simulink model "dynamic_model_soft_robot"  (R2018a)
settings: Solver=ode4  StartTime=0.0  StopTime=t_span  FixedStep=dt  RelTol=1e-3
values from neighbouring files (symbols this model uses):
  alpha0 = 0    [data_simulate_srm_dynamic_model.m]
  c1 = 0.12    [data_simulate_srm_dynamic_model.m]
  c2 = 5.93e-7    (= 5.93e-07)    [data_simulate_srm_dynamic_model.m]
  c3 = 5.93e-7    (= 5.93e-07)    [data_simulate_srm_dynamic_model.m]
  d0 = 0.0644    [data_simulate_srm_dynamic_model.m]
  dq_0 = [0; 0; 500]    [data_simulate_srm_dynamic_model.m]
  dt = 1.00e-03    (= 0.001)    [data_simulate_srm_dynamic_model.m]    (also in simulateSoftRobot.m)
  g = 9.81    [data_simulate_srm_dynamic_model.m]    (also in simulateSoftRobot.m)
  m = 0.0494    [data_simulate_srm_dynamic_model.m]    (also in simulateSoftRobot.m)
  noise_ddq = 0*[1e-4, 1e-4, 1e-4]    [data_simulate_srm_dynamic_model.m]
  noise_dq = 0*[1e-4, 1e-4, 1e-4]    [data_simulate_srm_dynamic_model.m]
  noise_q = 0*[1e-6, 1e-1, 1e-1]    [data_simulate_srm_dynamic_model.m]
  p_true = [b1; b2; b3; b4; b5; b6]    [data_simulate_srm_dynamic_model.m]
  q_0 = [d0; 10; .1]    [data_simulate_srm_dynamic_model.m]
  r = 0.0235    [data_simulate_srm_dynamic_model.m]    (also in simulateSoftRobot.m = 0.02)
libraries: dspinverses x1
(part 2 of 3)

== matlab function dynamic_model_soft_robot/soft robotic manipulator dynamical model/Coreoilis matrix  ==
  data: q input; y output; dq input; m parameter; r parameter
function y = fcn(q,dq,m,r)

l = q(1);
kappa_x = q(2);
kappa_y1 = q(3);

dl = dq(1);
dkappa_x = dq(2);
dkappa_y = dq(3);

C = zeros(3,3);

C(1,1) = (dl*(4.0*m*sin(l*(kappa_x^2 + kappa_y1^2)^(1/2)) - 4.0*l*m*cos(l*(kappa_x^2 + kappa_y1^2)^(1/2))*(kappa_x^2 + kappa_y1^2)^(1/2)))/(2*l^2*(kappa_x^2 + kappa_y1^2)^(3/2)) - (2.0*dkappa_x*kappa_x*m*(3.0*kappa_x^2*l*(kappa_x^2 + kappa_y1^2)^(1/2) - 3.0*kappa_x^2*sin(l*(kappa_x^2 + kappa_y1^2)^(1/2)) - 3.0*kappa_y1^2*sin(l*(kappa_x^2 + kappa_y1^2)^(1/2)) - 1.0*l*(kappa_x^2 + kappa_y1^2)^(3/2) + 3.0*kappa_y1^2*l*(kappa_x^2 + kappa_y1^2)^(1/2) + kappa_x^2*l*cos(l*(kappa_x^2 + kappa_y1^2)^(1/2))*(kappa_x^2 + kappa_y1^2)^(1/2) + kappa_y1^2*l*cos(l*(kappa_x^2 + kappa_y1^2)^(1/2))*(kappa_x^2 + kappa_y1^2)^(1/2)))/(l*(kappa_x^2 + kappa_y1^2)^(7/2)) - (2.0*dkappa_y*kappa_y1*m*(3.0*kappa_x^2*l*(kappa_x^2 + kappa_y1^2)^(1/2) - 3.0*kappa_x^2*sin(l*(kappa_x^2 + kappa_y1^2)^(1/2)) - 3.0*kappa_y1^2*sin(l*(kappa_x^2 + kappa_y1^2)^(1/2)) - 1.0*l*(kappa_x^2 + kappa_y1^2)^(3/2) + 3.0*kappa_y1^2*l*(kappa_x^2 + kappa_y1^2)^(1/2) + kappa_x^2*l*cos(l*(kappa_x^2 + kappa_y1^2)^(1/2))*(kappa_x^2 + kappa_y1^2)^(1/2) + kappa_y1^2*l*cos(l*(kappa_x^2 + kappa_y1^2)^(1/2))*(kappa_x^2 + kappa_y1^2)^(1/2)))/(l*(kappa_x^2 + kappa_y1^2)^(7/2));
C(1,2) = - (dkappa_y*(4.0*kappa_x*kappa_y1*m*sin(l*(kappa_x^2 + kappa_y1^2)^(1/2)) + 0.5*kappa_x*kappa_y1*m*sin(2.0*l*(kappa_x^2 + kappa_y1^2)^(1/2)) - 2.0*kappa_x*kappa_y1^3*m*r^2*sin(l*(kappa_x^2 + kappa_y1^2)^(1/2)) - 2.0*kappa_x^3*kappa_y1*m*r^2*sin(l*(kappa_x^2 + kappa_y1^2)^(1/2)) + 60.0*kappa_x*kappa_y1*l*m*sin(l*(kappa_x^2 + kappa_y1^2)^(1/2)) + 0.125*kappa_x*kappa_y1^3*m*r^2*sin(2.0*l*(kappa_x^2 + kappa_y1^2)^(1/2)) + 0.125*kappa_x^3*kappa_y1*m*r^2*sin(2.0*l*(kappa_x^2 + kappa_y1^2)^(1/2)) - 32.0*kappa_x*kappa_y1*l^2*m*(kappa_x^2 + kappa_y1^2)^(1/2) + 1.3333333333333333333333333333333*kappa_x*kappa_y1*l^3*m*(kappa_x^2 + kappa_y1^2)^(3/2) - 1.0*kappa_x*kappa_y1*l*m*cos(2.0*l*(kappa_x^2 + kappa_y1^2)^(1/2))*(kappa_x^2 + kappa_y1^2)^(1/2) - 28.0*kappa_x*kappa_y1*l^2*m*cos(l*(kappa_x^2 + kappa_y1^2)^(1/2))*(kappa_x^2 + kappa_y1^2)^(1/2) - 4.0*kappa_x*kappa_y1*l*m*cos(l*(kappa_x^2 + kappa_y1^2)^(1/2))*(kappa_x^2 + kappa_y1^2)^(1/2) + 0.33333333333333333333333333333333*kappa_x*kappa_y1^3*l^3*m*r^2*(kappa_x^2 + kappa_y1^2)^(3/2) + 0.33333333333333333333333333333333*kappa_x^3*kappa_y1*l^3*m*r^2*(kappa_x^2 + kappa_y1^2)^(3/2) - 4.0*kappa_x*kappa_y1*l^2*m*sin(l*(kappa_x^2 + kappa_y1^2)^(1/2))*(kappa_x^2 + kappa_y1^2) - 4*kappa_x*kappa_y1*l^3*m*sin(l*(kappa_x^2 + kappa_y1^2)^(1/2))*(kappa_x^2 + kappa_y1^2) + 2.0*kappa_x*kappa_y1^3*l*m*r^2*cos(l*(kappa_x^2 + kappa_y1^2)^(1/2))*(kappa_x^2 + kappa_y1^2)^(1/2) + 2.0*kappa_x^3*kappa_y1*l*m*r^2*cos(l*(kappa_x^2 + kappa_y1^2)^(1/2))*(kappa_x^2 + kappa_y1^2)^(1/2) - 0.25*kappa_x*kappa_y1^3*l*m*r^2*cos(2.0*l*(kappa_x^2 + kappa_y1^2)^(1/2))*(kappa_x^2 + kappa_y1^2)^(1/2) - 0.25*kappa_x^3*kappa_y1*l*m*r^2*cos(2.0*l*(kappa_x^2 + kappa_y1^2)^(1/2))*(kappa_x^2 + kappa_y1^2)^(1/2)))/(2*l^2*(kappa_x^2 + kappa_y1^2)^(7/2)) - (dkappa_x*(8.0*kappa_x^2*m*sin(l*(kappa_x^2 + kappa_y1^2)^(1/2)) + 4.0*kappa_y1^2*m*sin(l*(kappa_x^2 + kappa_y1^2)^(1/2)) - 0.5*kappa_y1^2*m*sin(2.0*l*(kappa_x^2 + kappa_y1^2)^(1/2)) + 8.0*l^2*m*(kappa_x^2 + kappa_y1^2)^(3/2) - 0.125*kappa_y1^4*m*r^2*sin(2.0*l*(kappa_x^2 + kappa_y1^2)^(1/2)) + 4*l^2*m*cos(l*(kappa_x^2 + kappa_y1^2)^(1/2))*(kappa_x^2 + kappa_y1^2)^(3/2) + 60.0*kappa_x^2*l*m*sin(l*(kappa_x^2 + kappa_y1^2)^(1/2)) - 32.0*kappa_x^2*l^2*m*(kappa_x^2 + kappa_y1^2)^(1/2) + 1.3333333333333333333333333333333*kappa_x^2*l^3*m*(kappa_x^2 + kappa_y1^2)^(3/2) - 12.0*l*m*sin(l*(kappa_x^2 + kappa_y1^2)^(1/2))*(kappa_x^2 + kappa_y1^2) + 2.0*kappa_y1^4*m*r^2*sin(l*(kappa_x^2 + kappa_y1^2)^(1/2)) - 0.125*kappa_x^2*kappa_y1^2*m*r^2*sin(2.0*l*(kappa_x^2 + kappa_y1^2)^(1/2)) + kappa_y1^2*l*m*cos(2.0*l*(kappa_x^2 + kappa_y1^2)^(1/2))*(kappa_x^2 + kappa_y1^2)^(1/2) - 28.0*kappa_x^2*l^2*m*cos(l*(kappa_x^2 + kappa_y1^2)^(1/2))*(kappa_x^2 + kappa_y1^2)^(1/2) + 0.33333333333333333333333333333333*kappa_x^4*l^3*m*r^2*(kappa_x^2 + kappa_y1^2)^(3/2) + 2.0*kappa_x^2*kappa_y1^2*m*r^2*sin(l*(kappa_x^2 + kappa_y1^2)^(1/2)) - 8.0*kappa_x^2*l*m*cos(l*(kappa_x^2 + kappa_y1^2)^(1/2))*(kappa_x^2 + kappa_y1^2)^(1/2) - 4.0*kappa_y1^2*l*m*cos(l*(kappa_x^2 + kappa_y1^2)^(1/2))*(kappa_x^2 + kappa_y1^2)^(1/2) - 4.0*kappa_x^2*l^2*m*sin(l*(kappa_x^2 + kappa_y1^2)^(1/2))*(kappa_x^2 + kappa_y1^2) - 4*kappa_x^2*l^3*m*sin(l*(kappa_x^2 + kappa_y1^2)^(1/2))*(kappa_x^2 + kappa_y1^2) + 0.33333333333333333333333333333333*kappa_x^2*kappa_y1^2*l^3*m*r^2*(kappa_x^2 + kappa_y1^2)^(3/2) - 2.0*kappa_y1^4*l*m*r^2*cos(l*(kappa_x^2 + kappa_y1^2)^(1/2))*(kappa_x^2 + kappa_y1^2)^(1/2) + 0.25*kappa_y1^4*l*m*r^2*cos(2.0*l*(kappa_x^2 + kappa_y1^2)^(1/2))*(kappa_x^2 + kappa_y1^2)^(1/2) - 2.0*kappa_x^2*kappa_y1^2*l*m*r^2*cos(l*(kappa_x^2 + kappa_y1^2)^(1/2))*(kappa_x^2 + kappa_y1^2)^(1/2) + 0.25*kappa_x^2*kappa_y1^2*l*m*r^2*cos(2.0*l*(kappa_x^2 + kappa_y1^2)^(1/2))*(kappa_x^2 + kappa_y1^2)^(1/2)))/(2*l^2*(kappa_x^2 + kappa_y1^2)^(7/2)) - (2.0*dl*kappa_x*m*(3.0*kappa_x^2*l*(kappa_x^2 + kappa_y1^2)^(1/2) - 3.0*kappa_x^2*sin(l*(kappa_x^2 + kappa_y1^2)^(1/2)) - 3.0*kappa_y1^2*sin(l*(kappa_x^2 + kappa_y1^2)^(1/2)) - 1.0*l*(kappa_x^2 + kappa_y1^2)^(3/2) + 3.0*kappa_y1^2*l*(kappa_x^2 + kappa_y1^2)^(1/2) + kappa_x^2*l*cos(l*(kappa_x^2 + kappa_y1^2)^(1/2))*(kappa_x^2 + kappa_y1^2)^(1/2) + kappa_y1^2*l*cos(l*(kappa_x^2 + kappa_y1^2)^(1/2))*(kappa_x^2 + kappa_y1^2)^(1/2)))/(l*(kappa_x^2 + kappa_y1^2)^(7/2));
C(1,3) = - (dkappa_x*(4.0*kappa_x*kappa_y1*m*sin(l*(kappa_x^2 + kappa_y1^2)^(1/2)) + 0.5*kappa_x*kappa_y1*m*sin(2.0*l*(kappa_x^2 + kappa_y1^2)^(1/2)) - 2.0*kappa_x*kappa_y1^3*m*r^2*sin(l*(kappa_x^2 + kappa_y1^2)^(1/2)) - 2.0*kappa_x^3*kappa_y1*m*r^2*sin(l*(kappa_x^2 + kappa_y1^2)^(1/2)) + 60.0*kappa_x*kappa_y1*l*m*sin(l*(kappa_x^2 + kappa_y1^2)^(1/2)) + 0.125*kappa_x*kappa_y1^3*m*r^2*sin(2.0*l*(kappa_x^2 + kappa_y1^2)^(1/2)) + 0.125*kappa_x^3*kappa_y1*m*r^2*sin(2.0*l*(kappa_x^2 + kappa_y1^2)^(1/2)) - 32.0*kappa_x*kappa_y1*l^2*m*(kappa_x^2 + kappa_y1^2)^(1/2) + 1.3333333333333333333333333333333*kappa_x*kappa_y1*l^3*m*(kappa_x^2 + kappa_y1^2)^(3/2) - 1.0*kappa_x*kappa_y1*l*m*cos(2.0*l*(kappa_x^2 + kappa_y1^2)^(1/2))*(kappa_x^2 + kappa_y1^2)^(1/2) - 28.0*kappa_x*kappa_y1*l^2*m*cos(l*(kappa_x^2 + kappa_y1^2)^(1/2))*(kappa_x^2 + kappa_y1^2)^(1/2) - 4.0*kappa_x*kappa_y1*l*m*cos(l*(kappa_x^2 + kappa_y1^2)^(1/2))*(kappa_x^2 + kappa_y1^2)^(1/2) + 0.33333333333333333333333333333333*kappa_x*kappa_y1^3*l^3*m*r^2*(kappa_x^2 + kappa_y1^2)^(3/2) + 0.33333333333333333333333333333333*kappa_x^3*kappa_y1*l^3*m*r^2*(kappa_x^2 + kappa_y1^2)^(3/2) - 4.0*kappa_x*kappa_y1*l^2*m*sin(l*(kappa_x^2 + kappa_y1^2)^(1/2))*(kappa_x^2 + kappa_y1^2) - 4*kappa_x*kappa_y1*l^3*m*sin(l*(kappa_x^2 + kappa_y1^2)^(1/2))*(kappa_x^2 + kappa_y1^2) + 2.0*kappa_x*kappa_y1^3*l*m*r^2*cos(l*(kappa_x^2 + kappa_y1^2)^(1/2))*(kappa_x^2 + kappa_y1^2)^(1/2) + 2.0*kappa_x^3*kappa_y1*l*m*r^2*cos(l*(kappa_x^2 + kappa_y1^2)^(1/2))*(kappa_x^2 + kappa_y1^2)^(1/2) - 0.25*kappa_x*kappa_y1^3*l*m*r^2*cos(2.0*l*(kappa_x^2 + kappa_y1^2)^(1/2))*(kappa_x^2 + kappa_y1^2)^(1/2) - 0.25*kappa_x^3*kappa_y1*l*m*r^2*cos(2.0*l*(kappa_x^2 + kappa_y1^2)^(1/2))*(kappa_x^2 + kappa_y1^2)^(1/2)))/(2*l^2*(kappa_x^2 + kappa_y1^2)^(7/2)) - (dkappa_y*(4.0*kappa_x^2*m*sin(l*(kappa_x^2 + kappa_y1^2)^(1/2)) + 8.0*kappa_y1^2*m*sin(l*(kappa_x^2 + kappa_y1^2)^(1/2)) - 0.5*kappa_x^2*m*sin(2.0*l*(kappa_x^2 + kappa_y1^2)^(1/2)) + 8.0*l^2*m*(kappa_x^2 + kappa_y1^2)^(3/2) - 0.125*kappa_x^4*m*r^2*sin(2.0*l*(kappa_x^2 + kappa_y1^2)^(1/2)) + 4*l^2*m*cos(l*(kappa_x^2 + kappa_y1^2)^(1/2))*(kappa_x^2 + kappa_y1^2)^(3/2) + 60.0*kappa_y1^2*l*m*sin(l*(kappa_x^2 + kappa_y1^2)^(1/2)) - 32.0*kappa_y1^2*l^2*m*(kappa_x^2 + kappa_y1^2)^(1/2) + 1.3333333333333333333333333333333*kappa_y1^2*l^3*m*(kappa_x^2 + kappa_y1^2)^(3/2) - 12.0*l*m*sin(l*(kappa_x^2 + kappa_y1^2)^(1/2))*(kappa_x^2 + kappa_y1^2) + 2.0*kappa_x^4*m*r^2*sin(l*(kappa_x^2 + kappa_y1^2)^(1/2)) - 0.125*kappa_x^2*kappa_y1^2*m*r^2*sin(2.0*l*(kappa_x^2 + kappa_y1^2)^(1/2)) + kappa_x^2*l*m*cos(2.0*l*(kappa_x^2 + kappa_y1^2)^(1/2))*(kappa_x^2 + kappa_y1^2)^(1/2) - 28.0*kappa_y1^2*l^2*m*cos(l*(kappa_x^2 + kappa_y1^2)^(1/2))*(kappa_x^2 + kappa_y1^2)^(1/2) + 0.33333333333333333333333333333333*kappa_y1^4*l^3*m*r^2*(kappa_x^2 + kappa_y1^2)^(3/2) + 2.0*kappa_x^2*kappa_y1^2*m*r^2*sin(l*(kappa_x^2 + kappa_y1^2)^(1/2)) - 4.0*kappa_x^2*l*m*cos(l*(kappa_x^2 + kappa_y1^2)^(1/2))*(kappa_x^2 + kappa_y1^2)^(1/2) - 8.0*kappa_y1^2*l*m*cos(l*(kappa_x^2 + kappa_y1^2)^(1/2))*(kappa_x^2 + kappa_y1^2)^(1/2) - 4.0*kappa_y1^2*l^2*m*sin(l*(kappa_x^2 + kappa_y1^2)^(1/2))*(kappa_x^2 + kappa_y1^2) - 4*kappa_y1^2*l^3*m*sin(l*(kappa_x^2 + kappa_y1^2)^(1/2))*(kappa_x^2 + kappa_y1^2) + 0.33333333333333333333333333333333*kappa_x^2*kappa_y1^2*l^3*m*r^2*(kappa_x^2 + kappa_y1^2)^(3/2) - 2.0*kappa_x^4*l*m*r^2*cos(l*(kappa_x^2 + kappa_y1^2)^(1/2))*(kappa_x^2 + kappa_y1^2)^(1/2) + 0.25*kappa_x^4*l*m*r^2*cos(2.0*l*(kappa_x^2 + kappa_y1^2)^(1/2))*(kappa_x^2 + kappa_y1^2)^(1/2) - 2.0*kappa_x^2*kappa_y1^2*l*m*r^2*cos(l*(kappa_x^2 + kappa_y1^2)^(1/2))*(kappa_x^2 + kappa_y1^2)^(1/2) + 0.25*kappa_x^2*kappa_y1^2*l*m*r^2*cos(2.0*l*(kappa_x^2 + kappa_y1^2)^(1/2))*(kappa_x^2 + kappa_y1^2)^(1/2)))/(2*l^2*(kappa_x^2 + kappa_y1^2)^(7/2)) - (2.0*dl*kappa_y1*m*(3.0*kappa_x^2*l*(kappa_x^2 + kappa_y1^2)^(1/2) - 3.0*kappa_x^2*sin(l*(kappa_x^2 + kappa_y1^2)^(1/2)) - 3.0*kappa_y1^2*sin(l*(kappa_x^2 + kappa_y1^2)^(1/2)) - 1.0*l*(kappa_x^2 + kappa_y1^2)^(3/2) + 3.0*kappa_y1^2*l*(kappa_x^2 + kappa_y1^2)^(1/2) + kappa_x^2*l*cos(l*(kappa_x^2 + kappa_y1^2)^(1/2))*(kappa_x^2 + kappa_y1^2)^(1/2) + kappa_y1^2*l*cos(l*(kappa_x^2 + kappa_y1^2)^(1/2))*(kappa_x^2 + kappa_y1^2)^(1/2)))/(l*(kappa_x^2 + kappa_y1^2)^(7/2));

C(2,1) = (dkappa_y*(4.0*kappa_x*kappa_y1*m*sin(l*(kappa_x^2 + kappa_y1^2)^(1/2)) + 0.5*kappa_x*kappa_y1*m*sin(2.0*l*(kappa_x^2 + kappa_y1^2)^(1/2)) - 2.0*kappa_x*kappa_y1^3*m*r^2*sin(l*(kappa_x^2 + kappa_y1^2)^(1/2)) - 2.0*kappa_x^3*kappa_y1*m*r^2*sin(l*(kappa_x^2 + kappa_y1^2)^(1/2)) + 0.125*kappa_x*kappa_y1^3*m*r^2*sin(2.0*l*(kappa_x^2 + kappa_y1^2)^(1/2)) + 0.125*kappa_x^3*kappa_y1*m*r^2*sin(2.0*l*(kappa_x^2 + kappa_y1^2)^(1/2)) + 1.3333333333333333333333333333333*kappa_x*kappa_y1*l^3*m*(kappa_x^2 + kappa_y1^2)^(3/2) - 1.0*kappa_x*kappa_y1*l*m*cos(2.0*l*(kappa_x^2 + kappa_y1^2)^(1/2))*(kappa_x^2 + kappa_y1^2)^(1/2) - 4.0*kappa_x*kappa_y1*l*m*cos(l*(kappa_x^2 + kappa_y1^2)^(1/2))*(kappa_x^2 + kappa_y1^2)^(1/2) + 0.33333333333333333333333333333333*kappa_x*kappa_y1^3*l^3*m*r^2*(kappa_x^2 + kappa_y1^2)^(3/2) + 0.33333333333333333333333333333333*kappa_x^3*kappa_y1*l^3*m*r^2*(kappa_x^2 + kappa_y1^2)^(3/2) - 4.0*kappa_x*kappa_y1*l^2*m*sin(l*(kappa_x^2 + kappa_y1^2)^(1/2))*(kappa_x^2 + kappa_y1^2) + 2.0*kappa_x*kappa_y1^3*l*m*r^2*cos(l*(kappa_x^2 + kappa_y1^2)^(1/2))*(kappa_x^2 + kappa_y1^2)^(1/2) + 2.0*kappa_x^3*kappa_y1*l*m*r^2*cos(l*(kappa_x^2 + kappa_y1^2)^(1/2))*(kappa_x^2 + kappa_y1^2)^(1/2) - 0.25*kappa_x*kappa_y1^3*l*m*r^2*cos(2.0*l*(kappa_x^2 + kappa_y1^2)^(1/2))*(kappa_x^2 + kappa_y1^2)^(1/2) - 0.25*kappa_x^3*kappa_y1*l*m*r^2*cos(2.0*l*(kappa_x^2 + kappa_y1^2)^(1/2))*(kappa_x^2 + kappa_y1^2)^(1/2)))/(2*l^2*(kappa_x^2 + kappa_y1^2)^(7/2)) + (dkappa_x*(8.0*kappa_x^2*m*sin(l*(kappa_x^2 + kappa_y1^2)^(1/2)) + 4.0*kappa_y1^2*m*sin(l*(kappa_x^2 + kappa_y1^2)^(1/2)) - 0.5*kappa_y1^2*m*sin(2.0*l*(kappa_x^2 + kappa_y1^2)^(1/2)) - 0.125*kappa_y1^4*m*r^2*sin(2.0*l*(kappa_x^2 + kappa_y1^2)^(1/2)) + 1.3333333333333333333333333333333*kappa_x^2*l^3*m*(kappa_x^2 + kappa_y1^2)^(3/2) + 2.0*kappa_y1^4*m*r^2*sin(l*(kappa_x^2 + kappa_y1^2)^(1/2)) - 0.125*kappa_x^2*kappa_y1^2*m*r^2*sin(2.0*l*(kappa_x^2 + kappa_y1^2)^(1/2)) + kappa_y1^2*l*m*cos(2.0*l*(kappa_x^2 + kappa_y1^2)^(1/2))*(kappa_x^2 + kappa_y1^2)^(1/2) + 0.33333333333333333333333333333333*kappa_x^4*l^3*m*r^2*(kappa_x^2 + kappa_y1^2)^(3/2) + 2.0*kappa_x^2*kappa_y1^2*m*r^2*sin(l*(kappa_x^2 + kappa_y1^2)^(1/2)) - 8.0*kappa_x^2*l*m*cos(l*(kappa_x^2 + kappa_y1^2)^(1/2))*(kappa_x^2 + kappa_y1^2)^(1/2) - 4.0*kappa_y1^2*l*m*cos(l*(kappa_x^2 + kappa_y1^2)^(1/2))*(kappa_x^2 + kappa_y1^2)^(1/2) - 4.0*kappa_x^2*l^2*m*sin(l*(kappa_x^2 + kappa_y1^2)^(1/2))*(kappa_x^2 + kappa_y1^2) + 0.33333333333333333333333333333333*kappa_x^2*kappa_y1^2*l^3*m*r^2*(kappa_x^2 + kappa_y1^2)^(3/2) - 2.0*kappa_y1^4*l*m*r^2*cos(l*(kappa_x^2 + kappa_y1^2)^(1/2))*(kappa_x^2 + kappa_y1^2)^(1/2) + 0.25*kappa_y1^4*l*m*r^2*cos(2.0*l*(kappa_x^2 + kappa_y1^2)^(1/2))*(kappa_x^2 + kappa_y1^2)^(1/2) - 2.0*kappa_x^2*kappa_y1^2*l*m*r^2*cos(l*(kappa_x^2 + kappa_y1^2)^(1/2))*(kappa_x^2 + kappa_y1^2)^(1/2) + 0.25*kappa_x^2*kappa_y1^2*l*m*r^2*cos(2.0*l*(kappa_x^2 + kappa_y1^2)^(1/2))*(kappa_x^2 + kappa_y1^2)^(1/2)))/(2*l^2*(kappa_x^2 + kappa_y1^2)^(7/2)) + (dl*(12.0*kappa_x^3*l^2*m*(kappa_x^2 + kappa_y1^2)^(1/2) - 20.0*kappa_x^3*l*m*sin(l*(kappa_x^2 + kappa_y1^2)^(1/2)) - 4.0*kappa_x*l^2*m*(kappa_x^2 + kappa_y1^2)^(3/2) - 12.0*kappa_x*m*sin(l*(kappa_x^2 + kappa_y1^2)^(1/2))*(kappa_x^2 + kappa_y1^2) - 20.0*kappa_x*kappa_y1^2*l*m*sin(l*(kappa_x^2 + kappa_y1^2)^(1/2)) + 12.0*kappa_x*kappa_y1^2*l^2*m*(kappa_x^2 + kappa_y1^2)^(1/2) + 8.0*kappa_x*l*m*sin(l*(kappa_x^2 + kappa_y1^2)^(1/2))*(kappa_x^2 + kappa_y1^2) + 4.0*kappa_x^3*l^2*m*cos(l*(kappa_x^2 + kappa_y1^2)^(1/2))*(kappa_x^2 + kappa_y1^2)^(1/2) + 12.0*kappa_x*l*m*cos(l*(kappa_x^2 + kappa_y1^2)^(1/2))*(kappa_x^2 + kappa_y1^2)^(3/2) + 4*kappa_x*l^2*m*sin(l*(kappa_x^2 + kappa_y1^2)^(1/2))*(kappa_x^2 + kappa_y1^2)^2 + 4.0*kappa_x*kappa_y1^2*l^2*m*cos(l*(kappa_x^2 + kappa_y1^2)^(1/2))*(kappa_x^2 + kappa_y1^2)^(1/2)))/(2*l^2*(kappa_x^2 + kappa_y1^2)^(7/2));
C(2,2) = (dl*(8.0*kappa_x^2*m*sin(l*(kappa_x^2 + kappa_y1^2)^(1/2)) + 4.0*kappa_y1^2*m*sin(l*(kappa_x^2 + kappa_y1^2)^(1/2)) - 0.5*kappa_y1^2*m*sin(2.0*l*(kappa_x^2 + kappa_y1^2)^(1/2)) - 0.125*kappa_y1^4*m*r^2*sin(2.0*l*(kappa_x^2 + kappa_y1^2)^(1/2)) + 1.3333333333333333333333333333333*kappa_x^2*l^3*m*(kappa_x^2 + kappa_y1^2)^(3/2) + 2.0*kappa_y1^4*m*r^2*sin(l*(kappa_x^2 + kappa_y1^2)^(1/2)) - 0.125*kappa_x^2*kappa_y1^2*m*r^2*sin(2.0*l*(kappa_x^2 + kappa_y1^2)^(1/2)) + kappa_y1^2*l*m*cos(2.0*l*(kappa_x^2 + kappa_y1^2)^(1/2))*(kappa_x^2 + kappa_y1^2)^(1/2) + 0.33333333333333333333333333333333*kappa_x^4*l^3*m*r^2*(kappa_x^2 + kappa_y1^2)^(3/2) + 2.0*kappa_x^2*kappa_y1^2*m*r^2*sin(l*(kappa_x^2 + kappa_y1^2)^(1/2)) - 8.0*kappa_x^2*l*m*cos(l*(kappa_x^2 + kappa_y1^2)^(1/2))*(kappa_x^2 + kappa_y1^2)^(1/2) - 4.0*kappa_y1^2*l*m*cos(l*(kappa_x^2 + kappa_y1^2)^(1/2))*(kappa_x^2 + kappa_y1^2)^(1/2) - 4.0*kappa_x^2*l^2*m*sin(l*(kappa_x^2 + kappa_y1^2)^(1/2))*(kappa_x^2 + kappa_y1^2) + 0.33333333333333333333333333333333*kappa_x^2*kappa_y1^2*l^3*m*r^2*(kappa_x^2 + kappa_y1^2)^(3/2) - 2.0*kappa_y1^4*l*m*r^2*cos(l*(kappa_x^2 + kappa_y1^2)^(1/2))*(kappa_x^2 + kappa_y1^2)^(1/2) + 0.25*kappa_y1^4*l*m*r^2*cos(2.0*l*(kappa_x^2 + kappa_y1^2)^(1/2))*(kappa_x^2 + kappa_y1^2)^(1/2) - 2.0*kappa_x^2*kappa_y1^2*l*m*r^2*cos(l*(kappa_x^2 + kappa_y1^2)^(1/2))*(kappa_x^2 + kappa_y1^2)^(1/2) + 0.25*kappa_x^2*kappa_y1^2*l*m*r^2*cos(2.0*l*(kappa_x^2 + kappa_y1^2)^(1/2))*(kappa_x^2 + kappa_y1^2)^(1/2)))/(2*l^2*(kappa_x^2 + kappa_y1^2)^(7/2)) - (5.0e-34*dkappa_y*(2.5e33*kappa_y1^3*m*sin(2.0*l*(kappa_x^2 + kappa_y1^2)^(1/2)) - 2.0e34*kappa_y1^3*m*sin(l*(kappa_x^2 + kappa_y1^2)^(1/2)) + 375000000000000000000000000000000.0*kappa_y1^5*m*r^2*sin(2.0*l*(kappa_x^2 + kappa_y1^2)^(1/2)) - 4.8e34*kappa_x^2*kappa_y1*m*sin(l*(kappa_x^2 + kappa_y1^2)^(1/2)) - 1.0e33*kappa_x^2*kappa_y1*m*sin(2.0*l*(kappa_x^2 + kappa_y1^2)^(1/2)) + 1.2e34*kappa_y1*l*m*(kappa_x^2 + kappa_y1^2)^(3/2) - 6.0e33*kappa_y1^5*m*r^2*sin(l*(kappa_x^2 + kappa_y1^2)^(1/2)) + 125000000000000000000000000000000.0*kappa_x^2*kappa_y1^3*m*r^2*sin(2.0*l*(kappa_x^2 + kappa_y1^2)^(1/2)) - 1.0e33*kappa_y1^3*l*m*cos(2.0*l*(kappa_x^2 + kappa_y1^2)^(1/2))*(kappa_x^2 + kappa_y1^2)^(1/2) + 2.6666666666666666666666666666667e33*kappa_x^2*kappa_y1*l^3*m*(kappa_x^2 + kappa_y1^2)^(3/2) + 5.0e33*kappa_y1^3*l*m*r^2*(kappa_x^2 + kappa_y1^2)^(3/2) + 1.5e33*kappa_y1^5*l*m*r^2*(kappa_x^2 + kappa_y1^2)^(1/2) + 4.0e33*kappa_x^4*kappa_y1*l^2*m*sin(l*(kappa_x^2 + kappa_y1^2)^(1/2)) + 4.0e33*kappa_x^4*kappa_y1*m*r^2*sin(l*(kappa_x^2 + kappa_y1^2)^(1/2)) - 250000000000000000000000000000000.0*kappa_x^4*kappa_y1*m*r^2*sin(2.0*l*(kappa_x^2 + kappa_y1^2)^(1/2)) + 4.0e33*kappa_x^2*kappa_y1^3*l^2*m*sin(l*(kappa_x^2 + kappa_y1^2)^(1/2)) + 6.0e33*kappa_x^2*kappa_y1*l*m*(kappa_x^2 + kappa_y1^2)^(1/2) - 2.0e33*kappa_x^2*kappa_y1^3*m*r^2*sin(l*(kappa_x^2 + kappa_y1^2)^(1/2)) - 3.0e33*kappa_y1*l*m*r^2*(kappa_x^2 + kappa_y1^2)^(5/2) + 4.0e33*kappa_y1^3*l*m*cos(l*(kappa_x^2 + kappa_y1^2)^(1/2))*(kappa_x^2 + kappa_y1^2)^(1/2) + 3.2e34*kappa_x^2*kappa_y1*l*m*cos(l*(kappa_x^2 + kappa_y1^2)^(1/2))*(kappa_x^2 + kappa_y1^2)^(1/2) + 666666666666666666666666666666677.0*kappa_x^2*kappa_y1^3*l^3*m*r^2*(kappa_x^2 + kappa_y1^2)^(3/2) - 500000000000000000000000000000000.0*kappa_x^2*kappa_y1*l*m*r^2*(kappa_x^2 + kappa_y1^2)^(3/2) + 2.0e33*kappa_y1^5*l*m*r^2*cos(l*(kappa_x^2 + kappa_y1^2)^(1/2))*(kappa_x^2 + kappa_y1^2)^(1/2) - 250000000000000000000000000000000.0*kappa_y1^5*l*m*r^2*cos(2.0*l*(kappa_x^2 + kappa_y1^2)^(1/2))*(kappa_x^2 + kappa_y1^2)^(1/2) + 1.5e33*kappa_x^2*kappa_y1^3*l*m*r^2*(kappa_x^2 + kappa_y1^2)^(1/2) - 333333333333333333333333333333333.0*kappa_x^2*kappa_y1*l^3*m*r^2*(kappa_x^2 + kappa_y1^2)^(5/2) + 666666666666666666666666666666677.0*kappa_x^4*kappa_y1*l^3*m*r^2*(kappa_x^2 + kappa_y1^2)^(3/2) + 2.0e33*kappa_x^2*kappa_y1^3*l*m*r^2*cos(l*(kappa_x^2 + kappa_y1^2)^(1/2))*(kappa_x^2 + kappa_y1^2)^(1/2) - 250000000000000000000000000000000.0*kappa_x^2*kappa_y1^3*l*m*r^2*cos(2.0*l*(kappa_x^2 + kappa_y1^2)^(1/2))*(kappa_x^2 + kappa_y1^2)^(1/2)))/(l*(kappa_x^2 + kappa_y1^2)^(9/2)) - (5.0e-34*dkappa_x*(6.0e33*kappa_x^3*l*m*(kappa_x^2 + kappa_y1^2)^(1/2) - 4.0e34*kappa_x^3*m*sin(l*(kappa_x^2 + kappa_y1^2)^(1/2)) - 1.3333333333333333333333333333333e33*kappa_x*l^3*m*(kappa_x^2 + kappa_y1^2)^(5/2) - 1.2e34*kappa_x*kappa_y1^2*m*sin(l*(kappa_x^2 + kappa_y1^2)^(1/2)) + 2.6666666666666666666666666666667e33*kappa_x^3*l^3*m*(kappa_x^2 + kappa_y1^2)^(3/2) + 3.5e33*kappa_x*kappa_y1^2*m*sin(2.0*l*(kappa_x^2 + kappa_y1^2)^(1/2)) + 4.0e33*kappa_x^5*l^2*m*sin(l*(kappa_x^2 + kappa_y1^2)^(1/2)) + 1.0e34*kappa_x*l*m*(kappa_x^2 + kappa_y1^2)^(3/2) + 625000000000000000000000000000000.0*kappa_x^3*kappa_y1^2*m*r^2*sin(2.0*l*(kappa_x^2 + kappa_y1^2)^(1/2)) - 1.0e34*kappa_x*kappa_y1^4*m*r^2*sin(l*(kappa_x^2 + kappa_y1^2)^(1/2)) - 8.0e33*kappa_x*l*m*cos(l*(kappa_x^2 + kappa_y1^2)^(1/2))*(kappa_x^2 + kappa_y1^2)^(3/2) - 666666666666666666666666666666677.0*kappa_x^3*l^3*m*r^2*(kappa_x^2 + kappa_y1^2)^(5/2) + 666666666666666666666666666666677.0*kappa_x^5*l^3*m*r^2*(kappa_x^2 + kappa_y1^2)^(3/2) + 625000000000000000000000000000000.0*kappa_x*kappa_y1^4*m*r^2*sin(2.0*l*(kappa_x^2 + kappa_y1^2)^(1/2)) + 4.0e33*kappa_x^3*kappa_y1^2*l^2*m*sin(l*(kappa_x^2 + kappa_y1^2)^(1/2)) - 1.0e34*kappa_x^3*kappa_y1^2*m*r^2*sin(l*(kappa_x^2 + kappa_y1^2)^(1/2)) + 3.2e34*kappa_x^3*l*m*cos(l*(kappa_x^2 + kappa_y1^2)^(1/2))*(kappa_x^2 + kappa_y1^2)^(1/2) + 4.0e33*kappa_x*kappa_y1^2*l*m*cos(l*(kappa_x^2 + kappa_y1^2)^(1/2))*(kappa_x^2 + kappa_y1^2)^(1/2) + 666666666666666666666666666666677.0*kappa_x^3*kappa_y1^2*l^3*m*r^2*(kappa_x^2 + kappa_y1^2)^(3/2) - 1.0e33*kappa_x*kappa_y1^2*l*m*cos(2.0*l*(kappa_x^2 + kappa_y1^2)^(1/2))*(kappa_x^2 + kappa_y1^2)^(1/2) + 5.5e33*kappa_x*kappa_y1^2*l*m*r^2*(kappa_x^2 + kappa_y1^2)^(3/2) + 1.5e33*kappa_x*kappa_y1^4*l*m*r^2*(kappa_x^2 + kappa_y1^2)^(1/2) + 1.5e33*kappa_x^3*kappa_y1^2*l*m*r^2*(kappa_x^2 + kappa_y1^2)^(1/2) - 333333333333333333333333333333333.0*kappa_x*kappa_y1^2*l^3*m*r^2*(kappa_x^2 + kappa_y1^2)^(5/2) + 2.0e33*kappa_x*kappa_y1^4*l*m*r^2*cos(l*(kappa_x^2 + kappa_y1^2)^(1/2))*(kappa_x^2 + kappa_y1^2)^(1/2) - 250000000000000000000000000000000.0*kappa_x*kappa_y1^4*l*m*r^2*cos(2.0*l*(kappa_x^2 + kappa_y1^2)^(1/2))*(kappa_x^2 + kappa_y1^2)^(1/2) + 2.0e33*kappa_x^3*kappa_y1^2*l*m*r^2*cos(l*(kappa_x^2 + kappa_y1^2)^(1/2))*(kappa_x^2 + kappa_y1^2)^(1/2) - 250000000000000000000000000000000.0*kappa_x^3*kappa_y1^2*l*m*r^2*cos(2.0*l*(kappa_x^2 + kappa_y1^2)^(1/2))*(kappa_x^2 + kappa_y1^2)^(1/2)))/(l*(kappa_x^2 + kappa_y1^2)^(9/2));
C(2,3) = (dkappa_y*(1.5*kappa_x^3*m*sin(2.0*l*(kappa_x^2 + kappa_y1^2)^(1/2)) - 28.0*kappa_x^3*m*sin(l*(kappa_x^2 + kappa_y1^2)^(1/2)) + 0.125*kappa_x^5*m*r^2*sin(2.0*l*(kappa_x^2 + kappa_y1^2)^(1/2)) + 1.3333333333333333333333333333333*kappa_x*l^3*m*(kappa_x^2 + kappa_y1^2)^(5/2) + 5.0*kappa_x*kappa_y1^2*m*sin(2.0*l*(kappa_x^2 + kappa_y1^2)^(1/2)) + 14.0*kappa_x*l*m*(kappa_x^2 + kappa_y1^2)^(3/2) - 2.0*kappa_x^5*m*r^2*sin(l*(kappa_x^2 + kappa_y1^2)^(1/2)) + 0.875*kappa_x^3*kappa_y1^2*m*r^2*sin(2.0*l*(kappa_x^2 + kappa_y1^2)^(1/2)) - 1.0*kappa_x^3*l*m*cos(2.0*l*(kappa_x^2 + kappa_y1^2)^(1/2))*(kappa_x^2 + kappa_y1^2)^(1/2) - 2.6666666666666666666666666666667*kappa_x*kappa_y1^2*l^3*m*(kappa_x^2 + kappa_y1^2)^(3/2) + 4.5*kappa_x^3*l*m*r^2*(kappa_x^2 + kappa_y1^2)^(3/2) + 1.5*kappa_x^5*l*m*r^2*(kappa_x^2 + kappa_y1^2)^(1/2) - 4.0*kappa_x*kappa_y1^4*l^2*m*sin(l*(kappa_x^2 + kappa_y1^2)^(1/2)) - 12.0*kappa_x*kappa_y1^4*m*r^2*sin(l*(kappa_x^2 + kappa_y1^2)^(1/2)) + 8.0*kappa_x*l*m*cos(l*(kappa_x^2 + kappa_y1^2)^(1/2))*(kappa_x^2 + kappa_y1^2)^(3/2) + 0.33333333333333333333333333333333*kappa_x^3*l^3*m*r^2*(kappa_x^2 + kappa_y1^2)^(5/2) + 0.75*kappa_x*kappa_y1^4*m*r^2*sin(2.0*l*(kappa_x^2 + kappa_y1^2)^(1/2)) - 4.0*kappa_x^3*kappa_y1^2*l^2*m*sin(l*(kappa_x^2 + kappa_y1^2)^(1/2)) - 6.0*kappa_x*kappa_y1^2*l*m*(kappa_x^2 + kappa_y1^2)^(1/2) - 14.0*kappa_x^3*kappa_y1^2*m*r^2*sin(l*(kappa_x^2 + kappa_y1^2)^(1/2)) - 6.0*kappa_x*l*m*r^2*(kappa_x^2 + kappa_y1^2)^(5/2) + 4.0*kappa_x^3*l*m*cos(l*(kappa_x^2 + kappa_y1^2)^(1/2))*(kappa_x^2 + kappa_y1^2)^(1/2) - 24.0*kappa_x*kappa_y1^2*l*m*cos(l*(kappa_x^2 + kappa_y1^2)^(1/2))*(kappa_x^2 + kappa_y1^2)^(1/2) - 0.66666666666666666666666666666667*kappa_x^3*kappa_y1^2*l^3*m*r^2*(kappa_x^2 + kappa_y1^2)^(3/2) - 2.0*kappa_x*kappa_y1^2*l*m*cos(2.0*l*(kappa_x^2 + kappa_y1^2)^(1/2))*(kappa_x^2 + kappa_y1^2)^(1/2) + 10.0*kappa_x*kappa_y1^2*l*m*r^2*(kappa_x^2 + kappa_y1^2)^(3/2) + 3.0*kappa_x*kappa_y1^4*l*m*r^2*(kappa_x^2 + kappa_y1^2)^(1/2) + 2.0*kappa_x^5*l*m*r^2*cos(l*(kappa_x^2 + kappa_y1^2)^(1/2))*(kappa_x^2 + kappa_y1^2)^(1/2) - 0.25*kappa_x^5*l*m*r^2*cos(2.0*l*(kappa_x^2 + kappa_y1^2)^(1/2))*(kappa_x^2 + kappa_y1^2)^(1/2) + 4.5*kappa_x^3*kappa_y1^2*l*m*r^2*(kappa_x^2 + kappa_y1^2)^(1/2) + 0.66666666666666666666666666666667*kappa_x*kappa_y1^2*l^3*m*r^2*(kappa_x^2 + kappa_y1^2)^(5/2) - 0.66666666666666666666666666666667*kappa_x*kappa_y1^4*l^3*m*r^2*(kappa_x^2 + kappa_y1^2)^(3/2) + 4.0*kappa_x*kappa_y1^4*l*m*r^2*cos(l*(kappa_x^2 + kappa_y1^2)^(1/2))*(kappa_x^2 + kappa_y1^2)^(1/2) - 0.5*kappa_x*kappa_y1^4*l*m*r^2*cos(2.0*l*(kappa_x^2 + kappa_y1^2)^(1/2))*(kappa_x^2 + kappa_y1^2)^(1/2) + 6.0*kappa_x^3*kappa_y1^2*l*m*r^2*cos(l*(kappa_x^2 + kappa_y1^2)^(1/2))*(kappa_x^2 + kappa_y1^2)^(1/2) - 0.75*kappa_x^3*kappa_y1^2*l*m*r^2*cos(2.0*l*(kappa_x^2 + kappa_y1^2)^(1/2))*(kappa_x^2 + kappa_y1^2)^(1/2)))/(2*l*(kappa_x^2 + kappa_y1^2)^(9/2)) - (5.0e-34*dkappa_x*(2.5e33*kappa_y1^3*m*sin(2.0*l*(kappa_x^2 + kappa_y1^2)^(1/2)) - 2.0e34*kappa_y1^3*m*sin(l*(kappa_x^2 + kappa_y1^2)^(1/2)) + 375000000000000000000000000000000.0*kappa_y1^5*m*r^2*sin(2.0*l*(kappa_x^2 + kappa_y1^2)^(1/2)) - 4.8e34*kappa_x^2*kappa_y1*m*sin(l*(kappa_x^2 + kappa_y1^2)^(1/2)) - 1.0e33*kappa_x^2*kappa_y1*m*sin(2.0*l*(kappa_x^2 + kappa_y1^2)^(1/2)) + 1.2e34*kappa_y1*l*m*(kappa_x^2 + kappa_y1^2)^(3/2) - 6.0e33*kappa_y1^5*m*r^2*sin(l*(kappa_x^2 + kappa_y1^2)^(1/2)) + 125000000000000000000000000000000.0*kappa_x^2*kappa_y1^3*m*r^2*sin(2.0*l*(kappa_x^2 + kappa_y1^2)^(1/2)) - 1.0e33*kappa_y1^3*l*m*cos(2.0*l*(kappa_x^2 + kappa_y1^2)^(1/2))*(kappa_x^2 + kappa_y1^2)^(1/2) + 2.6666666666666666666666666666667e33*kappa_x^2*kappa_y1*l^3*m*(kappa_x^2 + kappa_y1^2)^(3/2) + 5.0e33*kappa_y1^3*l*m*r^2*(kappa_x^2 + kappa_y1^2)^(3/2) + 1.5e33*kappa_y1^5*l*m*r^2*(kappa_x^2 + kappa_y1^2)^(1/2) + 4.0e33*kappa_x^4*kappa_y1*l^2*m*sin(l*(kappa_x^2 + kappa_y1^2)^(1/2)) + 4.0e33*kappa_x^4*kappa_y1*m*r^2*sin(l*(kappa_x^2 + kappa_y1^2)^(1/2)) - 250000000000000000000000000000000.0*kappa_x^4*kappa_y1*m*r^2*sin(2.0*l*(kappa_x^2 + kappa_y1^2)^(1/2)) + 4.0e33*kappa_x^2*kappa_y1^3*l^2*m*sin(l*(kappa_x^2 + kappa_y1^2)^(1/2)) + 6.0e33*kappa_x^2*kappa_y1*l*m*(kappa_x^2 + kappa_y1^2)^(1/2) - 2.0e33*kappa_x^2*kappa_y1^3*m*r^2*sin(l*(kappa_x^2 + kappa_y1^2)^(1/2)) - 3.0e33*kappa_y1*l*m*r^2*(kappa_x^2 + kappa_y1^2)^(5/2) + 4.0e33*kappa_y1^3*l*m*cos(l*(kappa_x^2 + kappa_y1^2)^(1/2))*(kappa_x^2 + kappa_y1^2)^(1/2) + 3.2e34*kappa_x^2*kappa_y1*l*m*cos(l*(kappa_x^2 + kappa_y1^2)^(1/2))*(kappa_x^2 + kappa_y1^2)^(1/2) + 666666666666666666666666666666677.0*kappa_x^2*kappa_y1^3*l^3*m*r^2*(kappa_x^2 + kappa_y1^2)^(3/2) - 500000000000000000000000000000000.0*kappa_x^2*kappa_y1*l*m*r^2*(kappa_x^2 + kappa_y1^2)^(3/2) + 2.0e33*kappa_y1^5*l*m*r^2*cos(l*(kappa_x^2 + kappa_y1^2)^(1/2))*(kappa_x^2 + kappa_y1^2)^(1/2) - 250000000000000000000000000000000.0*kappa_y1^5*l*m*r^2*cos(2.0*l*(kappa_x^2 + kappa_y1^2)^(1/2))*(kappa_x^2 + kappa_y1^2)^(1/2) + 1.5e33*kappa_x^2*kappa_y1^3*l*m*r^2*(kappa_x^2 + kappa_y1^2)^(1/2) - 333333333333333333333333333333333.0*kappa_x^2*kappa_y1*l^3*m*r^2*(kappa_x^2 + kappa_y1^2)^(5/2) + 666666666666666666666666666666677.0*kappa_x^4*kappa_y1*l^3*m*r^2*(kappa_x^2 + kappa_y1^2)^(3/2) + 2.0e33*kappa_x^2*kappa_y1^3*l*m*r^2*cos(l*(kappa_x^2 + kappa_y1^2)^(1/2))*(kappa_x^2 + kappa_y1^2)^(1/2) - 250000000000000000000000000000000.0*kappa_x^2*kappa_y1^3*l*m*r^2*cos(2.0*l*(kappa_x^2 + kappa_y1^2)^(1/2))*(kappa_x^2 + kappa_y1^2)^(1/2)))/(l*(kappa_x^2 + kappa_y1^2)^(9/2)) + (dl*(4.0*kappa_x*kappa_y1*m*sin(l*(kappa_x^2 + kappa_y1^2)^(1/2)) + 0.5*kappa_x*kappa_y1*m*sin(2.0*l*(kappa_x^2 + kappa_y1^2)^(1/2)) - 2.0*kappa_x*kappa_y1^3*m*r^2*sin(l*(kappa_x^2 + kappa_y1^2)^(1/2)) - 2.0*kappa_x^3*kappa_y1*m*r^2*sin(l*(kappa_x^2 + kappa_y1^2)^(1/2)) + 0.125*kappa_x*kappa_y1^3*m*r^2*sin(2.0*l*(kappa_x^2 + kappa_y1^2)^(1/2)) + 0.125*kappa_x^3*kappa_y1*m*r^2*sin(2.0*l*(kappa_x^2 + kappa_y1^2)^(1/2)) + 1.3333333333333333333333333333333*kappa_x*kappa_y1*l^3*m*(kappa_x^2 + kappa_y1^2)^(3/2) - 1.0*kappa_x*kappa_y1*l*m*cos(2.0*l*(kappa_x^2 + kappa_y1^2)^(1/2))*(kappa_x^2 + kappa_y1^2)^(1/2) - 4.0*kappa_x*kappa_y1*l*m*cos(l*(kappa_x^2 + kappa_y1^2)^(1/2))*(kappa_x^2 + kappa_y1^2)^(1/2) + 0.33333333333333333333333333333333*kappa_x*kappa_y1^3*l^3*m*r^2*(kappa_x^2 + kappa_y1^2)^(3/2) + 0.33333333333333333333333333333333*kappa_x^3*kappa_y1*l^3*m*r^2*(kappa_x^2 + kappa_y1^2)^(3/2) - 4.0*kappa_x*kappa_y1*l^2*m*sin(l*(kappa_x^2 + kappa_y1^2)^(1/2))*(kappa_x^2 + kappa_y1^2) + 2.0*kappa_x*kappa_y1^3*l*m*r^2*cos(l*(kappa_x^2 + kappa_y1^2)^(1/2))*(kappa_x^2 + kappa_y1^2)^(1/2) + 2.0*kappa_x^3*kappa_y1*l*m*r^2*cos(l*(kappa_x^2 + kappa_y1^2)^(1/2))*(kappa_x^2 + kappa_y1^2)^(1/2) - 0.25*kappa_x*kappa_y1^3*l*m*r^2*cos(2.0*l*(kappa_x^2 + kappa_y1^2)^(1/2))*(kappa_x^2 + kappa_y1^2)^(1/2) - 0.25*kappa_x^3*kappa_y1*l*m*r^2*cos(2.0*l*(kappa_x^2 + kappa_y1^2)^(1/2))*(kappa_x^2 + kappa_y1^2)^(1/2)))/(2*l^2*(kappa_x^2 + kappa_y1^2)^(7/2));
 
C(3,1) = (dkappa_x*(4.0*kappa_x*kappa_y1*m*sin(l*(kappa_x^2 + kappa_y1^2)^(1/2)) + 0.5*kappa_x*kappa_y1*m*sin(2.0*l*(kappa_x^2 + kappa_y1^2)^(1/2)) - 2.0*kappa_x*kappa_y1^3*m*r^2*sin(l*(kappa_x^2 + kappa_y1^2)^(1/2)) - 2.0*kappa_x^3*kappa_y1*m*r^2*sin(l*(kappa_x^2 + kappa_y1^2)^(1/2)) + 0.125*kappa_x*kappa_y1^3*m*r^2*sin(2.0*l*(kappa_x^2 + kappa_y1^2)^(1/2)) + 0.125*kappa_x^3*kappa_y1*m*r^2*sin(2.0*l*(kappa_x^2 + kappa_y1^2)^(1/2)) + 1.3333333333333333333333333333333*kappa_x*kappa_y1*l^3*m*(kappa_x^2 + kappa_y1^2)^(3/2) - 1.0*kappa_x*kappa_y1*l*m*cos(2.0*l*(kappa_x^2 + kappa_y1^2)^(1/2))*(kappa_x^2 + kappa_y1^2)^(1/2) - 4.0*kappa_x*kappa_y1*l*m*cos(l*(kappa_x^2 + kappa_y1^2)^(1/2))*(kappa_x^2 + kappa_y1^2)^(1/2) + 0.33333333333333333333333333333333*kappa_x*kappa_y1^3*l^3*m*r^2*(kappa_x^2 + kappa_y1^2)^(3/2) + 0.33333333333333333333333333333333*kappa_x^3*kappa_y1*l^3*m*r^2*(kappa_x^2 + kappa_y1^2)^(3/2) - 4.0*kappa_x*kappa_y1*l^2*m*sin(l*(kappa_x^2 + kappa_y1^2)^(1/2))*(kappa_x^2 + kappa_y1^2) + 2.0*kappa_x*kappa_y1^3*l*m*r^2*cos(l*(kappa_x^2 + kappa_y1^2)^(1/2))*(kappa_x^2 + kappa_y1^2)^(1/2) + 2.0*kappa_x^3*kappa_y1*l*m*r^2*cos(l*(kappa_x^2 + kappa_y1^2)^(1/2))*(kappa_x^2 + kappa_y1^2)^(1/2) - 0.25*kappa_x*kappa_y1^3*l*m*r^2*cos(2.0*l*(kappa_x^2 + kappa_y1^2)^(1/2))*(kappa_x^2 + kappa_y1^2)^(1/2) - 0.25*kappa_x^3*kappa_y1*l*m*r^2*cos(2.0*l*(kappa_x^2 + kappa_y1^2)^(1/2))*(kappa_x^2 + kappa_y1^2)^(1/2)))/(2*l^2*(kappa_x^2 + kappa_y1^2)^(7/2)) + (dkappa_y*(4.0*kappa_x^2*m*sin(l*(kappa_x^2 + kappa_y1^2)^(1/2)) + 8.0*kappa_y1^2*m*sin(l*(kappa_x^2 + kappa_y1^2)^(1/2)) - 0.5*kappa_x^2*m*sin(2.0*l*(kappa_x^2 + kappa_y1^2)^(1/2)) - 0.125*kappa_x^4*m*r^2*sin(2.0*l*(kappa_x^2 + kappa_y1^2)^(1/2)) + 1.3333333333333333333333333333333*kappa_y1^2*l^3*m*(kappa_x^2 + kappa_y1^2)^(3/2) + 2.0*kappa_x^4*m*r^2*sin(l*(kappa_x^2 + kappa_y1^2)^(1/2)) - 0.125*kappa_x^2*kappa_y1^2*m*r^2*sin(2.0*l*(kappa_x^2 + kappa_y1^2)^(1/2)) + kappa_x^2*l*m*cos(2.0*l*(kappa_x^2 + kappa_y1^2)^(1/2))*(kappa_x^2 + kappa_y1^2)^(1/2) + 0.33333333333333333333333333333333*kappa_y1^4*l^3*m*r^2*(kappa_x^2 + kappa_y1^2)^(3/2) + 2.0*kappa_x^2*kappa_y1^2*m*r^2*sin(l*(kappa_x^2 + kappa_y1^2)^(1/2)) - 4.0*kappa_x^2*l*m*cos(l*(kappa_x^2 + kappa_y1^2)^(1/2))*(kappa_x^2 + kappa_y1^2)^(1/2) - 8.0*kappa_y1^2*l*m*cos(l*(kappa_x^2 + kappa_y1^2)^(1/2))*(kappa_x^2 + kappa_y1^2)^(1/2) - 4.0*kappa_y1^2*l^2*m*sin(l*(kappa_x^2 + kappa_y1^2)^(1/2))*(kappa_x^2 + kappa_y1^2) + 0.33333333333333333333333333333333*kappa_x^2*kappa_y1^2*l^3*m*r^2*(kappa_x^2 + kappa_y1^2)^(3/2) - 2.0*kappa_x^4*l*m*r^2*cos(l*(kappa_x^2 + kappa_y1^2)^(1/2))*(kappa_x^2 + kappa_y1^2)^(1/2) + 0.25*kappa_x^4*l*m*r^2*cos(2.0*l*(kappa_x^2 + kappa_y1^2)^(1/2))*(kappa_x^2 + kappa_y1^2)^(1/2) - 2.0*kappa_x^2*kappa_y1^2*l*m*r^2*cos(l*(kappa_x^2 + kappa_y1^2)^(1/2))*(kappa_x^2 + kappa_y1^2)^(1/2) + 0.25*kappa_x^2*kappa_y1^2*l*m*r^2*cos(2.0*l*(kappa_x^2 + kappa_y1^2)^(1/2))*(kappa_x^2 + kappa_y1^2)^(1/2)))/(2*l^2*(kappa_x^2 + kappa_y1^2)^(7/2)) + (dl*(12.0*kappa_y1^3*l^2*m*(kappa_x^2 + kappa_y1^2)^(1/2) - 20.0*kappa_y1^3*l*m*sin(l*(kappa_x^2 + kappa_y1^2)^(1/2)) - 4.0*kappa_y1*l^2*m*(kappa_x^2 + kappa_y1^2)^(3/2) - 12.0*kappa_y1*m*sin(l*(kappa_x^2 + kappa_y1^2)^(1/2))*(kappa_x^2 + kappa_y1^2) - 20.0*kappa_x^2*kappa_y1*l*m*sin(l*(kappa_x^2 + kappa_y1^2)^(1/2)) + 12.0*kappa_x^2*kappa_y1*l^2*m*(kappa_x^2 + kappa_y1^2)^(1/2) + 8.0*kappa_y1*l*m*sin(l*(kappa_x^2 + kappa_y1^2)^(1/2))*(kappa_x^2 + kappa_y1^2) + 4.0*kappa_y1^3*l^2*m*cos(l*(kappa_x^2 + kappa_y1^2)^(1/2))*(kappa_x^2 + kappa_y1^2)^(1/2) + 12.0*kappa_y1*l*m*cos(l*(kappa_x^2 + kappa_y1^2)^(1/2))*(kappa_x^2 + kappa_y1^2)^(3/2) + 4*kappa_y1*l^2*m*sin(l*(kappa_x^2 + kappa_y1^2)^(1/2))*(kappa_x^2 + kappa_y1^2)^2 + 4.0*kappa_x^2*kappa_y1*l^2*m*cos(l*(kappa_x^2 + kappa_y1^2)^(1/2))*(kappa_x^2 + kappa_y1^2)^(1/2)))/(2*l^2*(kappa_x^2 + kappa_y1^2)^(7/2));
C(3,2) = (dkappa_x*(1.5*kappa_y1^3*m*sin(2.0*l*(kappa_x^2 + kappa_y1^2)^(1/2)) - 28.0*kappa_y1^3*m*sin(l*(kappa_x^2 + kappa_y1^2)^(1/2)) + 0.125*kappa_y1^5*m*r^2*sin(2.0*l*(kappa_x^2 + kappa_y1^2)^(1/2)) + 1.3333333333333333333333333333333*kappa_y1*l^3*m*(kappa_x^2 + kappa_y1^2)^(5/2) + 5.0*kappa_x^2*kappa_y1*m*sin(2.0*l*(kappa_x^2 + kappa_y1^2)^(1/2)) + 14.0*kappa_y1*l*m*(kappa_x^2 + kappa_y1^2)^(3/2) - 2.0*kappa_y1^5*m*r^2*sin(l*(kappa_x^2 + kappa_y1^2)^(1/2)) + 0.875*kappa_x^2*kappa_y1^3*m*r^2*sin(2.0*l*(kappa_x^2 + kappa_y1^2)^(1/2)) - 1.0*kappa_y1^3*l*m*cos(2.0*l*(kappa_x^2 + kappa_y1^2)^(1/2))*(kappa_x^2 + kappa_y1^2)^(1/2) - 2.6666666666666666666666666666667*kappa_x^2*kappa_y1*l^3*m*(kappa_x^2 + kappa_y1^2)^(3/2) + 4.5*kappa_y1^3*l*m*r^2*(kappa_x^2 + kappa_y1^2)^(3/2) + 1.5*kappa_y1^5*l*m*r^2*(kappa_x^2 + kappa_y1^2)^(1/2) - 4.0*kappa_x^4*kappa_y1*l^2*m*sin(l*(kappa_x^2 + kappa_y1^2)^(1/2)) - 12.0*kappa_x^4*kappa_y1*m*r^2*sin(l*(kappa_x^2 + kappa_y1^2)^(1/2)) + 8.0*kappa_y1*l*m*cos(l*(kappa_x^2 + kappa_y1^2)^(1/2))*(kappa_x^2 + kappa_y1^2)^(3/2) + 0.33333333333333333333333333333333*kappa_y1^3*l^3*m*r^2*(kappa_x^2 + kappa_y1^2)^(5/2) + 0.75*kappa_x^4*kappa_y1*m*r^2*sin(2.0*l*(kappa_x^2 + kappa_y1^2)^(1/2)) - 4.0*kappa_x^2*kappa_y1^3*l^2*m*sin(l*(kappa_x^2 + kappa_y1^2)^(1/2)) - 6.0*kappa_x^2*kappa_y1*l*m*(kappa_x^2 + kappa_y1^2)^(1/2) - 14.0*kappa_x^2*kappa_y1^3*m*r^2*sin(l*(kappa_x^2 + kappa_y1^2)^(1/2)) - 6.0*kappa_y1*l*m*r^2*(kappa_x^2 + kappa_y1^2)^(5/2) + 4.0*kappa_y1^3*l*m*cos(l*(kappa_x^2 + kappa_y1^2)^(1/2))*(kappa_x^2 + kappa_y1^2)^(1/2) - 24.0*kappa_x^2*kappa_y1*l*m*cos(l*(kappa_x^2 + kappa_y1^2)^(1/2))*(kappa_x^2 + kappa_y1^2)^(1/2) - 0.66666666666666666666666666666667*kappa_x^2*kappa_y1^3*l^3*m*r^2*(kappa_x^2 + kappa_y1^2)^(3/2) - 2.0*kappa_x^2*kappa_y1*l*m*cos(2.0*l*(kappa_x^2 + kappa_y1^2)^(1/2))*(kappa_x^2 + kappa_y1^2)^(1/2) + 10.0*kappa_x^2*kappa_y1*l*m*r^2*(kappa_x^2 + kappa_y1^2)^(3/2) + 3.0*kappa_x^4*kappa_y1*l*m*r^2*(kappa_x^2 + kappa_y1^2)^(1/2) + 2.0*kappa_y1^5*l*m*r^2*cos(l*(kappa_x^2 + kappa_y1^2)^(1/2))*(kappa_x^2 + kappa_y1^2)^(1/2) - 0.25*kappa_y1^5*l*m*r^2*cos(2.0*l*(kappa_x^2 + kappa_y1^2)^(1/2))*(kappa_x^2 + kappa_y1^2)^(1/2) + 4.5*kappa_x^2*kappa_y1^3*l*m*r^2*(kappa_x^2 + kappa_y1^2)^(1/2) + 0.66666666666666666666666666666667*kappa_x^2*kappa_y1*l^3*m*r^2*(kappa_x^2 + kappa_y1^2)^(5/2) - 0.66666666666666666666666666666667*kappa_x^4*kappa_y1*l^3*m*r^2*(kappa_x^2 + kappa_y1^2)^(3/2) + 4.0*kappa_x^4*kappa_y1*l*m*r^2*cos(l*(kappa_x^2 + kappa_y1^2)^(1/2))*(kappa_x^2 + kappa_y1^2)^(1/2) - 0.5*kappa_x^4*kappa_y1*l*m*r^2*cos(2.0*l*(kappa_x^2 + kappa_y1^2)^(1/2))*(kappa_x^2 + kappa_y1^2)^(1/2) + 6.0*kappa_x^2*kappa_y1^3*l*m*r^2*cos(l*(kappa_x^2 + kappa_y1^2)^(1/2))*(kappa_x^2 + kappa_y1^2)^(1/2) - 0.75*kappa_x^2*kappa_y1^3*l*m*r^2*cos(2.0*l*(kappa_x^2 + kappa_y1^2)^(1/2))*(kappa_x^2 + kappa_y1^2)^(1/2)))/(2*l*(kappa_x^2 + kappa_y1^2)^(9/2)) - (5.0e-34*dkappa_y*(2.5e33*kappa_x^3*m*sin(2.0*l*(kappa_x^2 + kappa_y1^2)^(1/2)) - 2.0e34*kappa_x^3*m*sin(l*(kappa_x^2 + kappa_y1^2)^(1/2)) + 375000000000000000000000000000000.0*kappa_x^5*m*r^2*sin(2.0*l*(kappa_x^2 + kappa_y1^2)^(1/2)) - 4.8e34*kappa_x*kappa_y1^2*m*sin(l*(kappa_x^2 + kappa_y1^2)^(1/2)) - 1.0e33*kappa_x*kappa_y1^2*m*sin(2.0*l*(kappa_x^2 + kappa_y1^2)^(1/2)) + 1.2e34*kappa_x*l*m*(kappa_x^2 + kappa_y1^2)^(3/2) - 6.0e33*kappa_x^5*m*r^2*sin(l*(kappa_x^2 + kappa_y1^2)^(1/2)) + 125000000000000000000000000000000.0*kappa_x^3*kappa_y1^2*m*r^2*sin(2.0*l*(kappa_x^2 + kappa_y1^2)^(1/2)) - 1.0e33*kappa_x^3*l*m*cos(2.0*l*(kappa_x^2 + kappa_y1^2)^(1/2))*(kappa_x^2 + kappa_y1^2)^(1/2) + 2.6666666666666666666666666666667e33*kappa_x*kappa_y1^2*l^3*m*(kappa_x^2 + kappa_y1^2)^(3/2) + 5.0e33*kappa_x^3*l*m*r^2*(kappa_x^2 + kappa_y1^2)^(3/2) + 1.5e33*kappa_x^5*l*m*r^2*(kappa_x^2 + kappa_y1^2)^(1/2) + 4.0e33*kappa_x*kappa_y1^4*l^2*m*sin(l*(kappa_x^2 + kappa_y1^2)^(1/2)) + 4.0e33*kappa_x*kappa_y1^4*m*r^2*sin(l*(kappa_x^2 + kappa_y1^2)^(1/2)) - 250000000000000000000000000000000.0*kappa_x*kappa_y1^4*m*r^2*sin(2.0*l*(kappa_x^2 + kappa_y1^2)^(1/2)) + 4.0e33*kappa_x^3*kappa_y1^2*l^2*m*sin(l*(kappa_x^2 + kappa_y1^2)^(1/2)) + 6.0e33*kappa_x*kappa_y1^2*l*m*(kappa_x^2 + kappa_y1^2)^(1/2) - 2.0e33*kappa_x^3*kappa_y1^2*m*r^2*sin(l*(kappa_x^2 + kappa_y1^2)^(1/2)) - 3.0e33*kappa_x*l*m*r^2*(kappa_x^2 + kappa_y1^2)^(5/2) + 4.0e33*kappa_x^3*l*m*cos(l*(kappa_x^2 + kappa_y1^2)^(1/2))*(kappa_x^2 + kappa_y1^2)^(1/2) + 3.2e34*kappa_x*kappa_y1^2*l*m*cos(l*(kappa_x^2 + kappa_y1^2)^(1/2))*(kappa_x^2 + kappa_y1^2)^(1/2) + 666666666666666666666666666666677.0*kappa_x^3*kappa_y1^2*l^3*m*r^2*(kappa_x^2 + kappa_y1^2)^(3/2) - 500000000000000000000000000000000.0*kappa_x*kappa_y1^2*l*m*r^2*(kappa_x^2 + kappa_y1^2)^(3/2) + 2.0e33*kappa_x^5*l*m*r^2*cos(l*(kappa_x^2 + kappa_y1^2)^(1/2))*(kappa_x^2 + kappa_y1^2)^(1/2) - 250000000000000000000000000000000.0*kappa_x^5*l*m*r^2*cos(2.0*l*(kappa_x^2 + kappa_y1^2)^(1/2))*(kappa_x^2 + kappa_y1^2)^(1/2) + 1.5e33*kappa_x^3*kappa_y1^2*l*m*r^2*(kappa_x^2 + kappa_y1^2)^(1/2) - 333333333333333333333333333333333.0*kappa_x*kappa_y1^2*l^3*m*r^2*(kappa_x^2 + kappa_y1^2)^(5/2) + 666666666666666666666666666666677.0*kappa_x*kappa_y1^4*l^3*m*r^2*(kappa_x^2 + kappa_y1^2)^(3/2) + 2.0e33*kappa_x^3*kappa_y1^2*l*m*r^2*cos(l*(kappa_x^2 + kappa_y1^2)^(1/2))*(kappa_x^2 + kappa_y1^2)^(1/2) - 250000000000000000000000000000000.0*kappa_x^3*kappa_y1^2*l*m*r^2*cos(2.0*l*(kappa_x^2 + kappa_y1^2)^(1/2))*(kappa_x^2 + kappa_y1^2)^(1/2)))/(l*(kappa_x^2 + kappa_y1^2)^(9/2)) + (dl*(4.0*kappa_x*kappa_y1*m*sin(l*(kappa_x^2 + kappa_y1^2)^(1/2)) + 0.5*kappa_x*kappa_y1*m*sin(2.0*l*(kappa_x^2 + kappa_y1^2)^(1/2)) - 2.0*kappa_x*kappa_y1^3*m*r^2*sin(l*(kappa_x^2 + kappa_y1^2)^(1/2)) - 2.0*kappa_x^3*kappa_y1*m*r^2*sin(l*(kappa_x^2 + kappa_y1^2)^(1/2)) + 0.125*kappa_x*kappa_y1^3*m*r^2*sin(2.0*l*(kappa_x^2 + kappa_y1^2)^(1/2)) + 0.125*kappa_x^3*kappa_y1*m*r^2*sin(2.0*l*(kappa_x^2 + kappa_y1^2)^(1/2)) + 1.3333333333333333333333333333333*kappa_x*kappa_y1*l^3*m*(kappa_x^2 + kappa_y1^2)^(3/2) - 1.0*kappa_x*kappa_y1*l*m*cos(2.0*l*(kappa_x^2 + kappa_y1^2)^(1/2))*(kappa_x^2 + kappa_y1^2)^(1/2) - 4.0*kappa_x*kappa_y1*l*m*cos(l*(kappa_x^2 + kappa_y1^2)^(1/2))*(kappa_x^2 + kappa_y1^2)^(1/2) + 0.33333333333333333333333333333333*kappa_x*kappa_y1^3*l^3*m*r^2*(kappa_x^2 + kappa_y1^2)^(3/2) + 0.33333333333333333333333333333333*kappa_x^3*kappa_y1*l^3*m*r^2*(kappa_x^2 + kappa_y1^2)^(3/2) - 4.0*kappa_x*kappa_y1*l^2*m*sin(l*(kappa_x^2 + kappa_y1^2)^(1/2))*(kappa_x^2 + kappa_y1^2) + 2.0*kappa_x*kappa_y1^3*l*m*r^2*cos(l*(kappa_x^2 + kappa_y1^2)^(1/2))*(kappa_x^2 + kappa_y1^2)^(1/2) + 2.0*kappa_x^3*kappa_y1*l*m*r^2*cos(l*(kappa_x^2 + kappa_y1^2)^(1/2))*(kappa_x^2 + kappa_y1^2)^(1/2) - 0.25*kappa_x*kappa_y1^3*l*m*r^2*cos(2.0*l*(kappa_x^2 + kappa_y1^2)^(1/2))*(kappa_x^2 + kappa_y1^2)^(1/2) - 0.25*kappa_x^3*kappa_y1*l*m*r^2*cos(2.0*l*(kappa_x^2 + kappa_y1^2)^(1/2))*(kappa_x^2 + kappa_y1^2)^(1/2)))/(2*l^2*(kappa_x^2 + kappa_y1^2)^(7/2));  
C(3,3) = (dl*(4.0*kappa_x^2*m*sin(l*(kappa_x^2 + kappa_y1^2)^(1/2)) + 8.0*kappa_y1^2*m*sin(l*(kappa_x^2 + kappa_y1^2)^(1/2)) - 0.5*kappa_x^2*m*sin(2.0*l*(kappa_x^2 + kappa_y1^2)^(1/2)) - 0.125*kappa_x^4*m*r^2*sin(2.0*l*(kappa_x^2 + kappa_y1^2)^(1/2)) + 1.3333333333333333333333333333333*kappa_y1^2*l^3*m*(kappa_x^2 + kappa_y1^2)^(3/2) + 2.0*kappa_x^4*m*r^2*sin(l*(kappa_x^2 + kappa_y1^2)^(1/2)) - 0.125*kappa_x^2*kappa_y1^2*m*r^2*sin(2.0*l*(kappa_x^2 + kappa_y1^2)^(1/2)) + kappa_x^2*l*m*cos(2.0*l*(kappa_x^2 + kappa_y1^2)^(1/2))*(kappa_x^2 + kappa_y1^2)^(1/2) + 0.33333333333333333333333333333333*kappa_y1^4*l^3*m*r^2*(kappa_x^2 + kappa_y1^2)^(3/2) + 2.0*kappa_x^2*kappa_y1^2*m*r^2*sin(l*(kappa_x^2 + kappa_y1^2)^(1/2)) - 4.0*kappa_x^2*l*m*cos(l*(kappa_x^2 + kappa_y1^2)^(1/2))*(kappa_x^2 + kappa_y1^2)^(1/2) - 8.0*kappa_y1^2*l*m*cos(l*(kappa_x^2 + kappa_y1^2)^(1/2))*(kappa_x^2 + kappa_y1^2)^(1/2) - 4.0*kappa_y1^2*l^2*m*sin(l*(kappa_x^2 + kappa_y1^2)^(1/2))*(kappa_x^2 + kappa_y1^2) + 0.33333333333333333333333333333333*kappa_x^2*kappa_y1^2*l^3*m*r^2*(kappa_x^2 + kappa_y1^2)^(3/2) - 2.0*kappa_x^4*l*m*r^2*cos(l*(kappa_x^2 + kappa_y1^2)^(1/2))*(kappa_x^2 + kappa_y1^2)^(1/2) + 0.25*kappa_x^4*l*m*r^2*cos(2.0*l*(kappa_x^2 + kappa_y1^2)^(1/2))*(kappa_x^2 + kappa_y1^2)^(1/2) - 2.0*kappa_x^2*kappa_y1^2*l*m*r^2*cos(l*(kappa_x^2 + kappa_y1^2)^(1/2))*(kappa_x^2 + kappa_y1^2)^(1/2) + 0.25*kappa_x^2*kappa_y1^2*l*m*r^2*cos(2.0*l*(kappa_x^2 + kappa_y1^2)^(1/2))*(kappa_x^2 + kappa_y1^2)^(1/2)))/(2*l^2*(kappa_x^2 + kappa_y1^2)^(7/2)) - (5.0e-34*dkappa_x*(2.5e33*kappa_x^3*m*sin(2.0*l*(kappa_x^2 + kappa_y1^2)^(1/2)) - 2.0e34*kappa_x^3*m*sin(l*(kappa_x^2 + kappa_y1^2)^(1/2)) + 375000000000000000000000000000000.0*kappa_x^5*m*r^2*sin(2.0*l*(kappa_x^2 + kappa_y1^2)^(1/2)) - 4.8e34*kappa_x*kappa_y1^2*m*sin(l*(kappa_x^2 + kappa_y1^2)^(1/2)) - 1.0e33*kappa_x*kappa_y1^2*m*sin(2.0*l*(kappa_x^2 + kappa_y1^2)^(1/2)) + 1.2e34*kappa_x*l*m*(kappa_x^2 + kappa_y1^2)^(3/2) - 6.0e33*kappa_x^5*m*r^2*sin(l*(kappa_x^2 + kappa_y1^2)^(1/2)) + 125000000000000000000000000000000.0*kappa_x^3*kappa_y1^2*m*r^2*sin(2.0*l*(kappa_x^2 + kappa_y1^2)^(1/2)) - 1.0e33*kappa_x^3*l*m*cos(2.0*l*(kappa_x^2 + kappa_y1^2)^(1/2))*(kappa_x^2 + kappa_y1^2)^(1/2) + 2.6666666666666666666666666666667e33*kappa_x*kappa_y1^2*l^3*m*(kappa_x^2 + kappa_y1^2)^(3/2) + 5.0e33*kappa_x^3*l*m*r^2*(kappa_x^2 + kappa_y1^2)^(3/2) + 1.5e33*kappa_x^5*l*m*r^2*(kappa_x^2 + kappa_y1^2)^(1/2) + 4.0e33*kappa_x*kappa_y1^4*l^2*m*sin(l*(kappa_x^2 + kappa_y1^2)^(1/2)) + 4.0e33*kappa_x*kappa_y1^4*m*r^2*sin(l*(kappa_x^2 + kappa_y1^2)^(1/2)) - 250000000000000000000000000000000.0*kappa_x*kappa_y1^4*m*r^2*sin(2.0*l*(kappa_x^2 + kappa_y1^2)^(1/2)) + 4.0e33*kappa_x^3*kappa_y1^2*l^2*m*sin(l*(kappa_x^2 + kappa_y1^2)^(1/2)) + 6.0e33*kappa_x*kappa_y1^2*l*m*(kappa_x^2 + kappa_y1^2)^(1/2) - 2.0e33*kappa_x^3*kappa_y1^2*m*r^2*sin(l*(kappa_x^2 + kappa_y1^2)^(1/2)) - 3.0e33*kappa_x*l*m*r^2*(kappa_x^2 + kappa_y1^2)^(5/2) + 4.0e33*kappa_x^3*l*m*cos(l*(kappa_x^2 + kappa_y1^2)^(1/2))*(kappa_x^2 + kappa_y1^2)^(1/2) + 3.2e34*kappa_x*kappa_y1^2*l*m*cos(l*(kappa_x^2 + kappa_y1^2)^(1/2))*(kappa_x^2 + kappa_y1^2)^(1/2) + 666666666666666666666666666666677.0*kappa_x^3*kappa_y1^2*l^3*m*r^2*(kappa_x^2 + kappa_y1^2)^(3/2) - 500000000000000000000000000000000.0*kappa_x*kappa_y1^2*l*m*r^2*(kappa_x^2 + kappa_y1^2)^(3/2) + 2.0e33*kappa_x^5*l*m*r^2*cos(l*(kappa_x^2 + kappa_y1^2)^(1/2))*(kappa_x^2 + kappa_y1^2)^(1/2) - 250000000000000000000000000000000.0*kappa_x^5*l*m*r^2*cos(2.0*l*(kappa_x^2 + kappa_y1^2)^(1/2))*(kappa_x^2 + kappa_y1^2)^(1/2) + 1.5e33*kappa_x^3*kappa_y1^2*l*m*r^2*(kappa_x^2 + kappa_y1^2)^(1/2) - 333333333333333333333333333333333.0*kappa_x*kappa_y1^2*l^3*m*r^2*(kappa_x^2 + kappa_y1^2)^(5/2) + 666666666666666666666666666666677.0*kappa_x*kappa_y1^4*l^3*m*r^2*(kappa_x^2 + kappa_y1^2)^(3/2) + 2.0e33*kappa_x^3*kappa_y1^2*l*m*r^2*cos(l*(kappa_x^2 + kappa_y1^2)^(1/2))*(kappa_x^2 + kappa_y1^2)^(1/2) - 250000000000000000000000000000000.0*kappa_x^3*kappa_y1^2*l*m*r^2*cos(2.0*l*(kappa_x^2 + kappa_y1^2)^(1/2))*(kappa_x^2 + kappa_y1^2)^(1/2)))/(l*(kappa_x^2 + kappa_y1^2)^(9/2)) - (5.0e-34*dkappa_y*(6.0e33*kappa_y1^3*l*m*(kappa_x^2 + kappa_y1^2)^(1/2) - 4.0e34*kappa_y1^3*m*sin(l*(kappa_x^2 + kappa_y1^2)^(1/2)) - 1.3333333333333333333333333333333e33*kappa_y1*l^3*m*(kappa_x^2 + kappa_y1^2)^(5/2) - 1.2e34*kappa_x^2*kappa_y1*m*sin(l*(kappa_x^2 + kappa_y1^2)^(1/2)) + 2.6666666666666666666666666666667e33*kappa_y1^3*l^3*m*(kappa_x^2 + kappa_y1^2)^(3/2) + 3.5e33*kappa_x^2*kappa_y1*m*sin(2.0*l*(kappa_x^2 + kappa_y1^2)^(1/2)) + 4.0e33*kappa_y1^5*l^2*m*sin(l*(kappa_x^2 + kappa_y1^2)^(1/2)) + 1.0e34*kappa_y1*l*m*(kappa_x^2 + kappa_y1^2)^(3/2) + 625000000000000000000000000000000.0*kappa_x^2*kappa_y1^3*m*r^2*sin(2.0*l*(kappa_x^2 + kappa_y1^2)^(1/2)) - 1.0e34*kappa_x^4*kappa_y1*m*r^2*sin(l*(kappa_x^2 + kappa_y1^2)^(1/2)) - 8.0e33*kappa_y1*l*m*cos(l*(kappa_x^2 + kappa_y1^2)^(1/2))*(kappa_x^2 + kappa_y1^2)^(3/2) - 666666666666666666666666666666677.0*kappa_y1^3*l^3*m*r^2*(kappa_x^2 + kappa_y1^2)^(5/2) + 666666666666666666666666666666677.0*kappa_y1^5*l^3*m*r^2*(kappa_x^2 + kappa_y1^2)^(3/2) + 625000000000000000000000000000000.0*kappa_x^4*kappa_y1*m*r^2*sin(2.0*l*(kappa_x^2 + kappa_y1^2)^(1/2)) + 4.0e33*kappa_x^2*kappa_y1^3*l^2*m*sin(l*(kappa_x^2 + kappa_y1^2)^(1/2)) - 1.0e34*kappa_x^2*kappa_y1^3*m*r^2*sin(l*(kappa_x^2 + kappa_y1^2)^(1/2)) + 3.2e34*kappa_y1^3*l*m*cos(l*(kappa_x^2 + kappa_y1^2)^(1/2))*(kappa_x^2 + kappa_y1^2)^(1/2) + 4.0e33*kappa_x^2*kappa_y1*l*m*cos(l*(kappa_x^2 + kappa_y1^2)^(1/2))*(kappa_x^2 + kappa_y1^2)^(1/2) + 666666666666666666666666666666677.0*kappa_x^2*kappa_y1^3*l^3*m*r^2*(kappa_x^2 + kappa_y1^2)^(3/2) - 1.0e33*kappa_x^2*kappa_y1*l*m*cos(2.0*l*(kappa_x^2 + kappa_y1^2)^(1/2))*(kappa_x^2 + kappa_y1^2)^(1/2) + 5.5e33*kappa_x^2*kappa_y1*l*m*r^2*(kappa_x^2 + kappa_y1^2)^(3/2) + 1.5e33*kappa_x^4*kappa_y1*l*m*r^2*(kappa_x^2 + kappa_y1^2)^(1/2) + 1.5e33*kappa_x^2*kappa_y1^3*l*m*r^2*(kappa_x^2 + kappa_y1^2)^(1/2) - 333333333333333333333333333333333.0*kappa_x^2*kappa_y1*l^3*m*r^2*(kappa_x^2 + kappa_y1^2)^(5/2) + 2.0e33*kappa_x^4*kappa_y1*l*m*r^2*cos(l*(kappa_x^2 + kappa_y1^2)^(1/2))*(kappa_x^2 + kappa_y1^2)^(1/2) - 250000000000000000000000000000000.0*kappa_x^4*kappa_y1*l*m*r^2*cos(2.0*l*(kappa_x^2 + kappa_y1^2)^(1/2))*(kappa_x^2 + kappa_y1^2)^(1/2) + 2.0e33*kappa_x^2*kappa_y1^3*l*m*r^2*cos(l*(kappa_x^2 + kappa_y1^2)^(1/2))*(kappa_x^2 + kappa_y1^2)^(1/2) - 250000000000000000000000000000000.0*kappa_x^2*kappa_y1^3*l*m*r^2*cos(2.0*l*(kappa_x^2 + kappa_y1^2)^(1/2))*(kappa_x^2 + kappa_y1^2)^(1/2)))/(l*(kappa_x^2 + kappa_y1^2)^(9/2));


y = C;
